simulink subsystem "Kalman_Filter"  (R2024a)
settings: Solver=VariableStepAuto  StartTime=0.0  StopTime=10.0  RelTol=1e-3
undefined symbols (not defined in the file): B, initial, L, MaxCurr, MaxCurr2, MinCurr1, MinCurr2, StateGain, xd
settings Model: Creator=Bocchio  LastModifiedBy=Bocchio

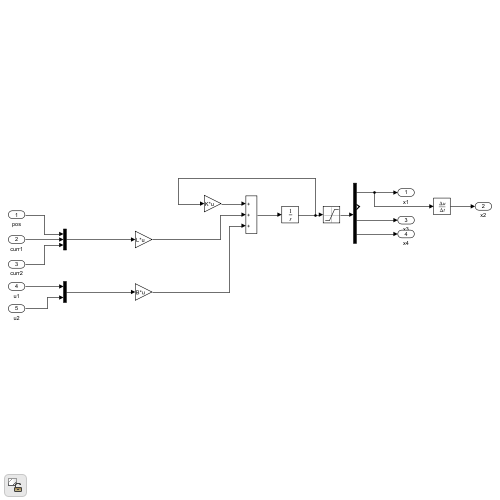
[thumbnail: Simulink's stored preview of the top-level diagram]
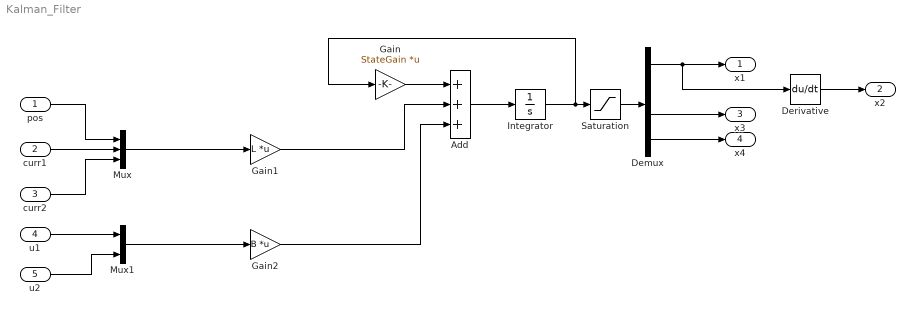
== system Kalman_Filter ==
  pos : Inport
  curr1 : Inport  Port=2
  curr2 : Inport  Port=3
  u1 : Inport  Port=4
  u2 : Inport  Port=5
  Add : Sum  Inputs=+++
  Demux : Demux
  Derivative : Derivative
  Gain : Gain  Gain=StateGain  Multiplication=Matrix(K*u)
  Gain1 : Gain  Gain=L  Multiplication=Matrix(K*u)
  Gain2 : Gain  Gain=B  Multiplication=Matrix(K*u)
  Integrator : Integrator  InitialCondition=[initial 0 MinCurr1 MinCurr2]
  Mux : Mux  Inputs=3
  Mux1 : Mux  Inputs=2
  Saturation : Saturate  UpperLimit=[xd inf MaxCurr MaxCurr2]  LowerLimit=[0 -inf MinCurr1 MinCurr2]
  x1 : Outport
  x2 : Outport  Port=2
  x3 : Outport  Port=3
  x4 : Outport  Port=4
  wires:
  Gain/1 -> Add/1
  Add/1 -> Integrator/1
  curr1/1 -> Mux/2
  pos/1 -> Mux/1
  curr2/1 -> Mux/3
  Mux/1 -> Gain1/1
  u1/1 -> Mux1/1
  u2/1 -> Mux1/2
  Mux1/1 -> Gain2/1
  Gain1/1 -> Add/2
  Gain2/1 -> Add/3
  Demux/1 -> x1/1, Derivative/1
  Demux/3 -> x3/1
  Demux/4 -> x4/1
  Saturation/1 -> Demux/1
  Integrator/1 -> Saturation/1, Gain/1
  Derivative/1 -> x2/1
